simulink model "ScalarCalculator"  (R2021a)
settings: Solver=FixedStepDiscrete  StartTime=0.0  StopTime=10.0  RelTol=1e-3  EnableMultiTasking=on
settings Model: Creator=Karim  LastModifiedBy=Karim
settings DataIOCC: ReturnWorkspaceOutputs=off
settings OptimizationCC: DefaultParameterBehavior=Inlined  InlineInvariantSignals=on  EnableMemcpy=off  LifeSpan=1  EfficientTunableParamExpr=on
settings DebuggingCC: UnderspecifiedInitializationDetection=Classic  MergeDetectMultiDrivingBlocksExec=none  SFMachineParentedDataDiag=warning  ArithmeticOperatorsInVariantConditions=warning
settings ModelReferenceCC: PropagateSignalLabelsOutOfModel=off
settings SFSimCC: MATLABDynamicMemAlloc=off  CustomCodeUndefinedFunction=UseInterfaceOnly
settings RTWCC: SystemTargetFile=ert.tlc  GenCodeOnly=on  TemplateMakefile=ert_default_tmf  GenerateReport=on  IncludeHyperlinkInReport=on  LaunchReport=on  GenerateTraceInfo=on  GenerateTraceReport=on  GenerateTraceReportSl=on  GenerateTraceReportSf=on  GenerateTraceReportEml=on
settings CodeAppCC: ForceParamTrailComments=on  IgnoreCustomStorageClasses=off  OperatorAnnotations=on  SimulinkDataObjDesc=on  SFDataObjDesc=on  MATLABFcnDesc=on  InsertBlockDesc=on  StateflowObjectComments=on  MATLABSourceComments=on
settings ERTTargetCC: MultiwordLength=2048  GenerateSampleERTMain=on  InlinedParameterPlacement=NonHierarchical  ERTCustomFileTemplate=example_file_process.tlc

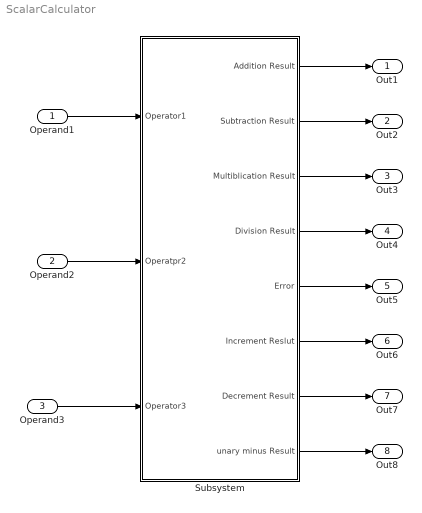
== system ScalarCalculator ==
  Operand1 : Inport
  Operand2 : Inport  Port=2
  Operand3 : Inport  Port=3
  Subsystem : Subsystem
  Out1 : Outport
  Out2 : Outport  Port=2
  Out3 : Outport  Port=3
  Out4 : Outport  Port=4
  Out5 : Outport  Port=5
  Out6 : Outport  Port=6
  Out7 : Outport  Port=7
  Out8 : Outport  Port=8
  wires:
  Operand2/1 -> Subsystem/2(Operatpr2)
  Subsystem/1(Addition Result) -> Out1/1
  Subsystem/2(Subtraction Result) -> Out2/1
  Subsystem/3(Multiblication Result) -> Out3/1
  Subsystem/4(Division Result) -> Out4/1
  Subsystem/5(Error) -> Out5/1
  Subsystem/6(Increment Reslut) -> Out6/1
  Subsystem/7(Decrement Result) -> Out7/1
  Subsystem/8(unary minus Result) -> Out8/1
  Operand1/1 -> Subsystem/1(Operator1)
  Operand3/1 -> Subsystem/3(Operator3)

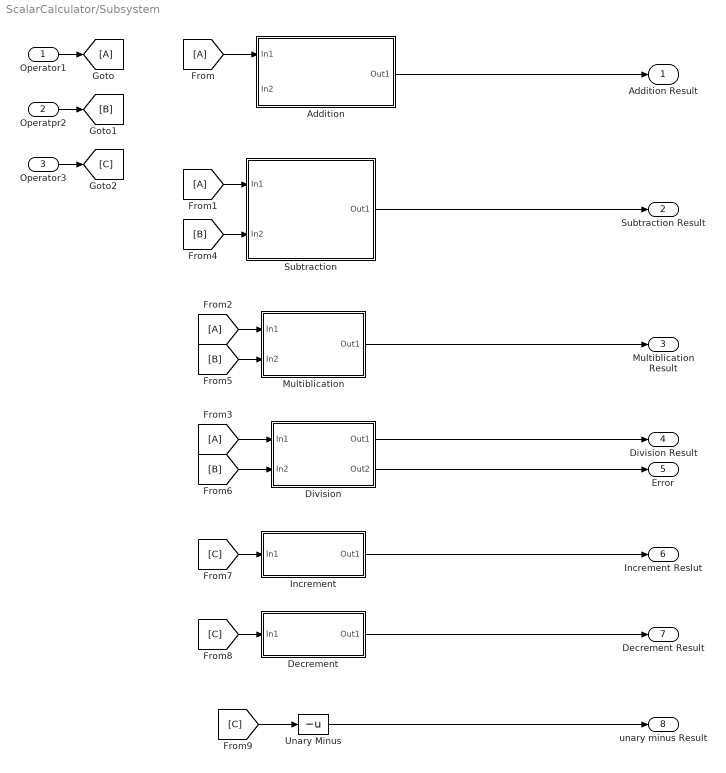
== system ScalarCalculator/Subsystem ==
  Operator1 : Inport
  Operatpr2 : Inport  Port=2
  Operator3 : Inport  Port=3
  Addition : Subsystem
  Decrement : Subsystem
  Division : Subsystem
  Increment : Subsystem
  Multiblication : Subsystem
  Subtraction : Subsystem
  Unary Minus : UnaryMinus
  Addition Result : Outport
  Subtraction Result : Outport  Port=2
  Multiblication Result : Outport  Port=3
  Division Result : Outport  Port=4
  Error : Outport  Port=5
  Increment Reslut : Outport  Port=6
  Decrement Result : Outport  Port=7
  unary minus Result : Outport  Port=8
  wires:
  Addition/1(Out1) -> Addition Result/1
  Subtraction/1(Out1) -> Subtraction Result/1
  Multiblication/1(Out1) -> Multiblication Result/1
  Division/1(Out1) -> Division Result/1
  Division/2(Out2) -> Error/1
  Increment/1(Out1) -> Increment Reslut/1
  Decrement/1(Out1) -> Decrement Result/1
  Unary Minus/1 -> unary minus Result/1
  Operator1/1 -> [A]
  [A] -> Addition/1(In1)
  [A] -> Division/1(In1)
  [A] -> Subtraction/1(In1)
  [A] -> Multiblication/1(In1)
  Operatpr2/1 -> [B]
  [B] -> Subtraction/2(In2)
  [B] -> Multiblication/2(In2)
  [B] -> Division/2(In2)
  Operator3/1 -> [C]
  [C] -> Increment/1(In1)
  [C] -> Decrement/1(In1)
  [C] -> Unary Minus/1

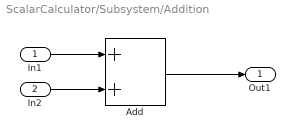
== system ScalarCalculator/Subsystem/Addition ==
  In1 : Inport
  In2 : Inport  Port=2
  Add : Sum
  Out1 : Outport
  wires:
  Add/1 -> Out1/1
  In1/1 -> Add/1
  In2/1 -> Add/2

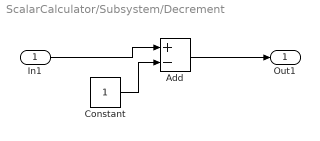
== system ScalarCalculator/Subsystem/Decrement ==
  In1 : Inport
  Add : Sum  Inputs=+-
  Constant : Constant
  Out1 : Outport
  wires:
  Constant/1 -> Add/2
  In1/1 -> Add/1
  Add/1 -> Out1/1

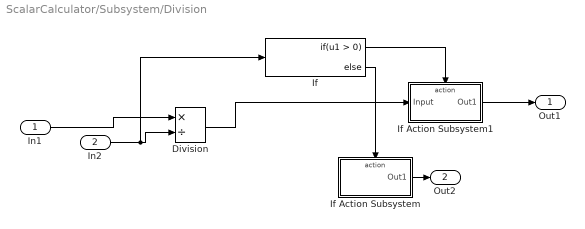
== system ScalarCalculator/Subsystem/Division ==
  In1 : Inport
  In2 : Inport  Port=2
  Division : Product  Inputs=*/
  If : If
  If Action Subsystem : Subsystem  TreatAsAtomicUnit=on
  If Action Subsystem1 : Subsystem  TreatAsAtomicUnit=on
  Out1 : Outport
  Out2 : Outport  Port=2
  wires:
  In1/1 -> Division/1
  In2/1 -> If/1, Division/2
  Division/1 -> If Action Subsystem1/1(Input)
  If/2 -> If Action Subsystem/Action
  If Action Subsystem/1(Out1) -> Out2/1
  If/1 -> If Action Subsystem1/Action
  If Action Subsystem1/1(Out1) -> Out1/1

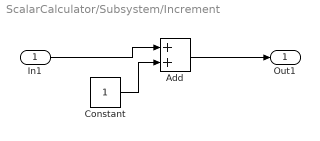
== system ScalarCalculator/Subsystem/Increment ==
  In1 : Inport
  Add : Sum
  Constant : Constant
  Out1 : Outport
  wires:
  Constant/1 -> Add/2
  In1/1 -> Add/1
  Add/1 -> Out1/1

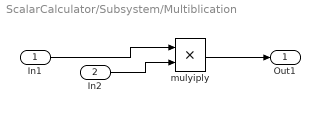
== system ScalarCalculator/Subsystem/Multiblication ==
  In1 : Inport
  In2 : Inport  Port=2
  mulyiply : Product  Inputs=**
  Out1 : Outport
  wires:
  In1/1 -> mulyiply/1
  In2/1 -> mulyiply/2
  mulyiply/1 -> Out1/1

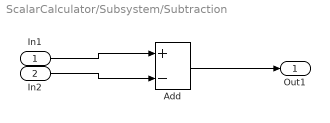
== system ScalarCalculator/Subsystem/Subtraction ==
  In1 : Inport
  In2 : Inport  Port=2
  Add : Sum  Inputs=+-
  Out1 : Outport
  wires:
  In1/1 -> Add/1
  In2/1 -> Add/2
  Add/1 -> Out1/1

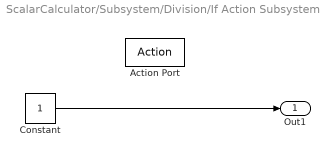
== system ScalarCalculator/Subsystem/Division/If Action Subsystem ==
  Action Port : ActionPort  ActionPortLabel=else
  Constant : Constant
  Out1 : Outport
  wires:
  Constant/1 -> Out1/1

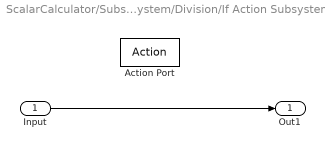
== system ScalarCalculator/Subsystem/Division/If Action Subsystem1 ==
  Input : Inport
  Action Port : ActionPort  ActionPortLabel=if(u1 > 0)
  Out1 : Outport
  wires:
  Input/1 -> Out1/1
